simulink model "JLN_Ballast_Tank_ver2"  (R2021a)
settings: Solver=VariableStepAuto  StartTime=0.0  StopTime=80  RelTol=1e-3
libraries: pid_lib x1
settings Model: Creator=naido  LastModifiedBy=naido

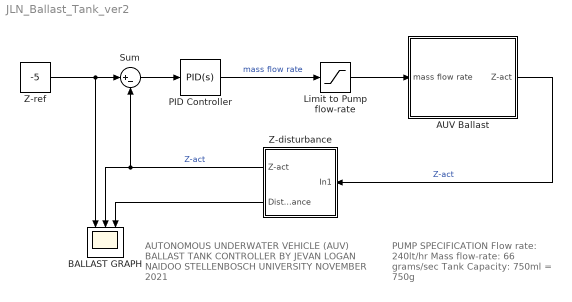
== system JLN_Ballast_Tank_ver2 ==
  note: PUMP SPECIFICATION
      |
      | Flow rate: 240lt/hr
      | Mass flow-rate: 66 grams/sec
      | Tank Capacity: 750ml = 750g
  note: AUTONOMOUS UNDERWATER VEHICLE (AUV)
      |
      | BALLAST TANK CONTROLLER
      |
      | BY JEVAN LOGAN NAIDOO
      | STELLENBOSCH UNIVERSITY
      | NOVEMBER 2021
  AUV Ballast : Subsystem
  BALLAST GRAPH : Scope  NumInputPorts=3
  Limit to Pump flow-rate : Saturate  UpperLimit=66  LowerLimit=-66
  PID Controller : pid_lib/PID Controller  Controller=PID  Form=Parallel  TimeDomain=Continuous-time  UseExternalTs=off  SampleTime=-1  IntegratorMethod=Forward Euler  FilterMethod=Forward Euler  ControllerParametersSource=internal  P=122.039157897355  I=21.5558012348095  D=23.1766203350516  UseFilter=on  N=3.646824066771  TunerSelectOption=Transfer Function Based (PID Tuner App)  InitialConditionSource=internal  InitialConditionForIntegrator=0  InitialConditionForFilter=0  DifferentiatorICPrevScaledInput=0  ExternalReset=none  TrackingMode=off  Kt=1  LimitOutput=off  SatLimitsSource=internal  UpperSaturationLimit=inf  LowerSaturationLimit=-inf  LinearizeAsGain=on  AntiWindupMode=none  Kb=1  POutMin=[]  POutMax=[]  IOutMin=[]  IOutMax=[]  DOutMin=[]  DOutMax=[]  NOutMin=[]  NOutMax=[]  SumOutMin=[]  SumOutMax=[]  SaturationOutMin=[]  SaturationOutMax=[]  PParamMin=[]  PParamMax=[]  IParamMin=[]  IParamMax=[]  DParamMin=[]  DParamMax=[]  NParamMin=[]  NParamMax=[]  KbParamMin=[]  KbParamMax=[]  KtParamMin=[]  KtParamMax=[]  KbOutMin=[]  KbOutMax=[]  KtOutMin=[]  KtOutMax=[]  IntegratorOutMin=[]  IntegratorOutMax=[]  FilterOutMin=[]  FilterOutMax=[]  SumI1OutMin=[]  SumI1OutMax=[]  SumI2OutMin=[]  SumI2OutMax=[]  SumI3OutMin=[]  SumI3OutMax=[]  SumI4OutMin=[]  SumI4OutMax=[]  SumDOutMin=[]  SumDOutMax=[]  DifferentiatorOutMin=[]  DifferentiatorOutMax=[]  FilterDiffOutCoefMin=[]  FilterDiffOutCoefMax=[]  ReciprocalOutMin=[]  ReciprocalOutMax=[]  SumDenOutMin=[]  SumDenOutMax=[]  SumNumOutMin=[]  SumNumOutMax=[]  DivideOutMin=[]  DivideOutMax=[]  UdiffTsProdOutMin=[]  UdiffTsProdOutMax=[]  NTsProdOutMin=[]  NTsProdOutMax=[]  UintegralTsProdOutMin=[]  UintegralTsProdOutMax=[]  UngainTsProdOutMin=[]  UngainTsProdOutMax=[]  IntegratorContinuousStateAttributes=''  IntegratorStateMustResolveToSignalObject=off  IntegratorRTWStateStorageClass=Auto  FilterContinuousStateAttributes=''  FilterStateMustResolveToSignalObject=off  FilterRTWStateStorageClass=Auto  ParallelPVariant=InternalParameters  IdealPVariant=Disabled  IVariant=InternalParameters  DVariant=InternalParameters  IntegratorVariant=Continuous  SatVariant=Disabled  AWVariant=Passthrough  PCopyVariant=Disabled  TRVariant=Disabled  FdbkBlocksVariant=Forward  IdealPFdbkVariant=Disabled  SatFdbkVariant=Disabled  DerivativeFilterVariant=ContFilter  NVariant=InternalParameters  NCopyVariant=Disabled  FilterICVariant=InternalICsFilter  IntegratorICVariant=InternalICs  ExternalResetVariant=Disabled  TRSumVariant=Passthrough  SumFdbkVariant=Disabled  SumVariant=Sum_PID  TsampFilterVariant=InternalTs  TsampNgainVariant=Passthrough  TsampIntegralVariant=Passthrough  ExternalSaturationOutDataTypeStr=Inherit: Same as second input
  Sum : Sum  Inputs=|+-
  Z-disturbance : Subsystem
  Z-ref : Constant  Value=-5
  wires:
  Sum/1 -> PID Controller/1
  Z-ref/1 -> BALLAST GRAPH/1, Sum/1
  AUV Ballast/1(Z-act) -> Z-disturbance/1(In1)  "Z-act"
  PID Controller/1 -> Limit to Pump flow-rate/1  "mass flow rate"
  Z-disturbance/1(Z-act) -> Sum/2, BALLAST GRAPH/2  "Z-act"
  Z-disturbance/2(Disturbance) -> BALLAST GRAPH/3
  Limit to Pump flow-rate/1 -> AUV Ballast/1(mass flow rate)

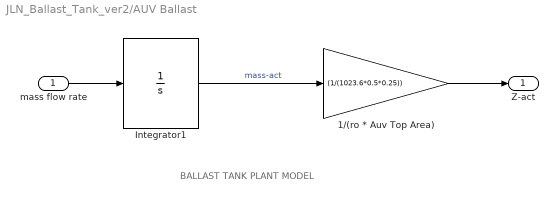
== system JLN_Ballast_Tank_ver2/AUV Ballast ==
  note: BALLAST TANK PLANT MODEL
  mass flow rate : Inport
  1/(ro * Auv Top Area) : Gain  Gain=(1/(1023.6*0.5*0.25))
  Integrator1 : Integrator
  Z-act : Outport
  wires:
  mass flow rate/1 -> Integrator1/1
  Integrator1/1 -> 1/(ro * Auv Top Area)/1  "mass-act"
  1/(ro * Auv Top Area)/1 -> Z-act/1

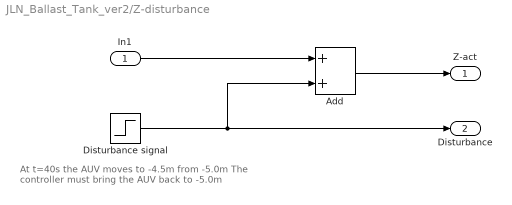
== system JLN_Ballast_Tank_ver2/Z-disturbance ==
  note: At t=40s the AUV moves to -4.5m from -5.0m
      | The controller must bring the AUV back to -5.0m
  In1 : Inport
  Add : Sum
  Disturbance signal : Step  Time=40  Before=-5  After=-4.5  SampleTime=0
  Z-act : Outport
  Disturbance : Outport  Port=2
  wires:
  Disturbance signal/1 -> Disturbance/1, Add/2
  In1/1 -> Add/1
  Add/1 -> Z-act/1
